simulink library "powerlib_extras"  (Simulink 6.0)
settings: Solver=ode45  SolverMode=SingleTasking  StartTime=0.0  StopTime=10.0  RelTol=1e-3
values from neighbouring files (symbols this model uses):
  Ts = get(handles.edit1,'string')    [powergui.m]
undefined symbols (not defined in the file or in its folder): Ac, Bc, Cc, Dc, Delay_discrete, dend, DiscIntNeverNeededParam, extra_sc, j, numd, test_alpha
libraries: powerlib2 x112, powerlib_extras x70, simulink_extras x25, simulink x12, powerlib_models x8
(part 5 of 9)

== system powerlib_extras/Discrete  Control Blocks/Discrete Monostable ==
  note: Discrete Monostable
  note: Silvano Casoria
      | Power System Simulation Laboratory
      | IREQ, Hydro-Quebc
  In : Inport  Port=1  LatchInput=off
  Constant2 : Constant  Value=-Ts
  Constant3 : Constant  Value=Ts
  Edge_Detector : Subsystem  mask(Discrete Edge Detector){model=EdgeDetect, ic=ic, Ts=Ts}
      mask prompts: model "Edge:"; ic "Input at t = -Ts:"; Ts "Sample time Ts:"
      mask help:
      | This block compares its present input to its previous input.
      |
      | If the input  is a logic signal (TRUE (1) or FALSE (0), the output is a one-step boolean signal TRUE  when  the specified edge (Rising, Falling or Either)  is detected.
      |
      | This block can also be used to detect the slope polarity of a continuous signal. For example, if the specified edge is  "Rising", the output is TRUE as long as the slope of the input signal is positive.
      |
      | The input value at time step preceeding t=0 is specified by the parameter "Input at t=-Ts"
      mask init: same as powerlib_extras/Control  Blocks/Edge Detector
      mask Display: plot(0,0,100,100, X1,Y1,X2,Y2,X3,Y3,X4,Y4);
  Logical Operator1 : Logic
  Logical Operator2 : Logic  Orientation=left  Operator=NOT  Inputs=1
  Relational Operator : RelationalOperator  Operator=>  InputSameDT=on
  Sum1 : Sum  Inputs=+-  SaturateOnIntegerOverflow=on  InputSameDT=on
  Switch : Switch  Threshold=0.5  SaturateOnIntegerOverflow=on  InputSameDT=on
  T_monostable : Constant  Value=t_mono
  Unit Delay : UnitDelay  Orientation=left  SampleTime=Ts
  delay : UnitDelay  Orientation=left  SampleTime=Ts
  Out : Outport
  wires:
  Sum1/1 -> Unit Delay/1, Relational Operator/1
  Unit Delay/1 -> Switch/3
  Constant3/1 -> Sum1/2
  Switch/1 -> Sum1/1
  T_monostable/1 -> Switch/1
  In/1 -> Edge_Detector/1(In)
  Relational Operator/1 -> delay/1, Out/1
  Logical Operator1/1 -> Switch/2
  delay/1 -> Logical Operator2/1
  Logical Operator2/1 -> Logical Operator1/1
  Edge_Detector/1(Out) -> Logical Operator1/2
  Constant2/1 -> Relational Operator/2

== system powerlib_extras/Discrete  Control Blocks/Discrete On/Off Delay ==
  note: Silvano Casoria
      | Power System Simulation Laboratory
      | IREQ, Hydro-Quebc
  note: Discrete On/Off Delay
  IN : Inport  Port=1  LatchInput=off
  Constant : Constant
  Constant1 : Constant  Value=delay
  Constant2 : Constant  Value=type_delay
  Data Type Conversion1 : DataTypeConversion  OutDataTypeMode=boolean  SaturateOnIntegerOverflow=on  RndMeth=Zero
  Logical Operator1 : Logic  Operator=OR
  Logical Operator2 : Logic  Operator=NOT  Inputs=1
  OFF Delay : Subsystem  TreatAsAtomicUnit=on
  ON Delay : Subsystem  TreatAsAtomicUnit=on
  Relational Operator1 : RelationalOperator  Operator===  InputSameDT=on
  OUT : Outport
  wires:
  Data Type Conversion1/1 -> ON Delay/1(IN), OFF Delay/1(IN)
  Constant/1 -> Relational Operator1/2
  Relational Operator1/1 -> ON Delay/Enable, Logical Operator2/1
  Constant2/1 -> Relational Operator1/1
  Logical Operator2/1 -> OFF Delay/Enable
  OFF Delay/1(OUT) -> Logical Operator1/2
  ON Delay/1(OUT) -> Logical Operator1/1
  Logical Operator1/1 -> OUT/1
  Constant1/1 -> ON Delay/2(DELAY), OFF Delay/2(DELAY)
  IN/1 -> Data Type Conversion1/1

== system powerlib_extras/Discrete  Control Blocks/Discrete PI Controller ==
  note: Pierre Giroux, Gilbert Sybille
      | Power System Simulation Laboratory
      | IREQ, Hydro-Quebc
  note: Discrete PID Controller
  Error : Inport  Port=1  LatchInput=off
  Discrete-Time Integrator : DiscreteIntegrator  InitialCondition=Init  SampleTime=Ts  LimitOutput=on  UpperSaturationLimit=UpperLimit  LowerSaturationLimit=LowerLimit  ICPrevOutput=DiscIntNeverNeededParam  ICPrevScaledInput=DiscIntNeverNeededParam
  Kp4 : Gain  Gain=Kp  SaturateOnIntegerOverflow=on
  Kp5 : Gain  Gain=Ki  SaturateOnIntegerOverflow=on
  Saturation2 : Saturate  UpperLimit=UpperLimit  LowerLimit=LowerLimit
  Sum6 : Sum  SaturateOnIntegerOverflow=on  InputSameDT=on
  Out : Outport  InitialOutput=0
  wires:
  Error/1 -> Kp4/1, Kp5/1
  Sum6/1 -> Saturation2/1
  Kp5/1 -> Discrete-Time Integrator/1
  Kp4/1 -> Sum6/1
  Discrete-Time Integrator/1 -> Sum6/2
  Saturation2/1 -> Out/1

== system powerlib_extras/Discrete  Control Blocks/Discrete PID Controller ==
  note: Discrete PID Controller
  note: Pierre Giroux, Gilbert Sybille
      | Power System Simulation Laboratory
      | IREQ, Hydro-Quebc
  Error : Inport  Port=1  LatchInput=off
  "Derivative " : DiscreteTransferFcn  Numerator=[2 -2]  Denominator=[Ts+2*TcD Ts-2*TcD]  SampleTime=Ts
  Discrete-Time Integrator : DiscreteIntegrator  InitialCondition=Init  SampleTime=Ts  LimitOutput=on  UpperSaturationLimit=UpperLimit  LowerSaturationLimit=LowerLimit  ICPrevOutput=DiscIntNeverNeededParam  ICPrevScaledInput=DiscIntNeverNeededParam
  Kp4 : Gain  Gain=Kp  SaturateOnIntegerOverflow=on
  Kp5 : Gain  Gain=Ki  SaturateOnIntegerOverflow=on
  Kp6 : Gain  Gain=Kd  SaturateOnIntegerOverflow=on
  Saturation2 : Saturate  UpperLimit=UpperLimit  LowerLimit=LowerLimit
  Sum6 : Sum  Inputs=+++  SaturateOnIntegerOverflow=on  InputSameDT=on
  Out : Outport  InitialOutput=0
  wires:
  Saturation2/1 -> Out/1
  "Derivative "/1 -> Sum6/3
  Discrete-Time Integrator/1 -> Sum6/2
  Kp4/1 -> Sum6/1
  Kp6/1 -> "Derivative "/1
  Kp5/1 -> Discrete-Time Integrator/1
  Sum6/1 -> Saturation2/1
  Error/1 -> Kp6/1, Kp5/1, Kp4/1

== system powerlib_extras/Discrete  Control Blocks/Discrete PWM Generator ==
  note: PWM Generator
  note: Pierre Giroux, Gilbert Sybille
      | Power System Laboratory, IREQ
      | Hydro-Quebec
  Signal(s) : Inport  Port=1  LatchInput=off
  BL4 : Logic  Operator=NOT  Inputs=1
  BL5 : Logic  Operator=NOT  Inputs=1
  Constant : Constant  Value=Internal_Phase
  Constant1 : Constant  Value=Internal
  Data Type  Conversion : DataTypeConversion  Orientation=down  OutDataTypeMode=double  SaturateOnIntegerOverflow=on  RndMeth=Zero
  Data Type  Conversion1 : DataTypeConversion  OutDataTypeMode=boolean  SaturateOnIntegerOverflow=on  RndMeth=Zero
  Data Type  Conversion2 : DataTypeConversion  OutDataTypeMode=boolean  SaturateOnIntegerOverflow=on  RndMeth=Zero
  Gain : Gain  Gain=2*pi*Freq  SaturateOnIntegerOverflow=on
  Gain2 : Gain  Gain=pi/180  SaturateOnIntegerOverflow=on
  Gain3 : Gain  Gain=-1  SaturateOnIntegerOverflow=on
  Mux : Mux  Inputs=2
  Mux1 : Mux  Inputs=2
  Mux2 : Mux  Inputs=2
  Product : Product  SaturateOnIntegerOverflow=on  InputSameDT=on
  Relational Operator : RelationalOperator  InputSameDT=on
  Relational Operator1 : RelationalOperator  InputSameDT=on
  Select1A : Selector  Elements=Select1_Elements  InputPortWidth=Select1_PortWidth
  Select1B : Selector  Elements=Select1_Elements  InputPortWidth=Select1_PortWidth
  Select3 : Selector  Elements=Select3_Elements  InputPortWidth=Select3_PortWidth
  Sum : Sum  Inputs=+++  SaturateOnIntegerOverflow=on  InputSameDT=on
  Switch : Switch  Threshold=0.5  SaturateOnIntegerOverflow=on  InputSameDT=on
  Triangle : simulink/Sources/Repeating Sequence  rep_seq_t=[0 1/Fc/4 3/Fc/4 1/Fc]  rep_seq_y=[0 -1 1 0]
  Trigonometric Function : Trigonometry
  m3 : Constant  Value=Phase
  m4 : Constant  Value=mIndex
  t : DigitalClock  SampleTime=Ts
  Pulses : Outport
  wires:
  Data Type  Conversion2/1 -> Mux1/1, BL5/1
  Relational Operator1/1 -> Data Type  Conversion2/1
  Data Type  Conversion1/1 -> Mux/1, BL4/1
  Relational Operator/1 -> Data Type  Conversion1/1
  Data Type  Conversion/1 -> Pulses/1
  Select3/1 -> Data Type  Conversion/1
  t/1 -> Gain/1
  Gain/1 -> Sum/1
  Gain2/1 -> Sum/2
  m3/1 -> Gain2/1
  Constant/1 -> Sum/3
  m4/1 -> Product/1
  Sum/1 -> Trigonometric Function/1
  Trigonometric Function/1 -> Product/2
  Signal(s)/1 -> Switch/3
  Constant1/1 -> Switch/2
  Product/1 -> Switch/1
  Triangle/1 -> Relational Operator/2, Relational Operator1/2
  Gain3/1 -> Relational Operator1/1
  BL4/1 -> Mux/2
  BL5/1 -> Mux1/2
  Mux/1 -> Select1A/1
  Mux1/1 -> Select1B/1
  Select1A/1 -> Mux2/1
  Select1B/1 -> Mux2/2
  Mux2/1 -> Select3/1
  Switch/1 -> Gain3/1, Relational Operator/1

== system powerlib_extras/Discrete  Control Blocks/Discrete Rate Limiter ==
  note: Delta(u)
  note: Beat Ronner
      | ABB Industrie AG
      | Turgi, Switzerland
  In : Inport  Port=1  LatchInput=off
  Saturation : Saturate  UpperLimit=UpperLimit  LowerLimit=LowerLimit
  Sum : Sum  Inputs=|++  SaturateOnIntegerOverflow=on  InputSameDT=on
  Sum1 : Sum  Inputs=|+-  SaturateOnIntegerOverflow=on  InputSameDT=on
  Unit  Delay : UnitDelay  Orientation=left  X0=Vinit  SampleTime=Ts
  Out : Outport
  wires:
  In/1 -> Sum1/1  "u"
  Sum1/1 -> Saturation/1
  Saturation/1 -> Sum/1  "Delta(u)_limit"
  Sum/1 -> Out/1, Unit  Delay/1  "y"
  Unit  Delay/1 -> Sum1/2, Sum/2  "y-1"

== system powerlib_extras/Discrete  Control Blocks/Discrete Sample & Hold ==
  note: Sample and Hold
  note: Silvano Casoria
      | Power System Simulation Laboratory
      | IREQ, Hydro-Quebc
  In : Inport  Port=1  LatchInput=off
  S : Inport  Port=2  LatchInput=off
  Switch : Switch  Threshold=0.5  SaturateOnIntegerOverflow=on  InputSameDT=on
  Unit Delay : UnitDelay  Orientation=left  X0=ic  SampleTime=Ts
  "   " : Outport  InitialOutput=0
  wires:
  Switch/1 -> Unit Delay/1, "   "/1
  Unit Delay/1 -> Switch/3
  In/1 -> Switch/1
  S/1 -> Switch/2

== system powerlib_extras/Discrete  Control Blocks/Discrete Shift Register ==
  u(k) : Inport  Port=1  LatchInput=off
  "S-Function " : S-Function  FunctionName=discreteNLastSamples  Parameters=NSamples,Ts,InitialValue
  Out : Outport
  wires:
  "S-Function "/1 -> Out/1
  u(k)/1 -> "S-Function "/1

== system powerlib_extras/Discrete  Control Blocks/Discrete Virtual PLL ==
  note: Discrete Virtual PLL
  note: Pierre Giroux, Gilbert Sybille
      | Power System Simulation Laboratory
      | IREQ, Hydro-Quebc
  Constant4 : Constant  Value=2*pi
  Deg->Rad : Gain  Gain=pi/180  SaturateOnIntegerOverflow=on
  Freq1 : Constant  Value=Freq
  Freq2 : Constant  Value=2*pi
  Initial Vd_Vq1 : Constant  Value=Phase
  Math Function : Math  Operator=mod  SaturateOnIntegerOverflow=on
  Mux : Mux  Inputs=2
  Product : Product  Inputs=***  SaturateOnIntegerOverflow=on  InputSameDT=on
  Sum : Sum  SaturateOnIntegerOverflow=on  InputSameDT=on
  Trigonometric Function : Trigonometry
  Trigonometric Function1 : Trigonometry  Operator=cos
  t : DigitalClock  SampleTime=Ts
  Freq : Outport
  Sin_Cos : Outport  Port=2
  wt : Outport  Port=3
  wires:
  Mux/1 -> Sin_Cos/1
  Trigonometric Function1/1 -> Mux/2
  Trigonometric Function/1 -> Mux/1
  Math Function/1 -> Trigonometric Function/1, Trigonometric Function1/1, wt/1
  Constant4/1 -> Math Function/2
  Product/1 -> Sum/1
  Initial Vd_Vq1/1 -> Deg->Rad/1
  Deg->Rad/1 -> Sum/2
  Freq1/1 -> Freq/1, Product/1
  Freq2/1 -> Product/3
  t/1 -> Product/2
  Sum/1 -> Math Function/1

== system powerlib_extras/Discrete  Control Blocks/Discrete  2nd-Order Filter ==
  In : Inport  Port=1  LatchInput=off
  Discrete State-Space : DiscreteStateSpace  A=Ad  B=Bd  C=Cd  D=Dd  X0=x0d  SampleTime=Ts
  Out : Outport  InitialOutput=0
  wires:
  In/1 -> Discrete State-Space/1
  Discrete State-Space/1 -> Out/1

== system powerlib_extras/Discrete  Control Blocks/Discrete  Butterworth Filter  ==
  In : Inport  Port=1  LatchInput=off
  Discrete State-Space : DiscreteStateSpace  A=Ad  B=Bd  C=Cd  D=Dd  X0=x0d  SampleTime=Ts
  Out : Outport  InitialOutput=0
  wires:
  In/1 -> Discrete State-Space/1
  Discrete State-Space/1 -> Out/1

== system powerlib_extras/Discrete  Control Blocks/Discrete 12-Pulse HVDC Control  ==
  note: Silvano Casoria
      | (Rev. 2001)
      | Power System Laboratory, IREQ
      | Hydro-Quebec
  note: Note 2 : gamma control is not implemented
  note: Note 1 : PLL is not simulated ; a fixed frequency is assumed
  note: Rect = 0
      | Inverter = 1
  note: 12-PULSE HVDC CONTROL
  Vabc (pu) : Inport  Port=1  LatchInput=off
  VdL (pu) : Inport  Port=2  LatchInput=off
  Id (pu) : Inport  Port=3  LatchInput=off
  Id_ref (pu) : Inport  Port=4  LatchInput=off
  Vd_ref (pu) : Inport  Port=5  LatchInput=off
  Block : Inport  Port=6  LatchInput=off
  ForcedAlpha : Inport  Port=7  LatchInput=off
  2nd order BP filters : Subsystem
  Alpha Control : Subsystem  mask{test_alpha=test_alpha, alpha_fix=alpha_fix}
      mask prompts: test_alpha "alpha control (0=normal; 1=constant alpha)"; alpha_fix "Constant alpha value (degrees) :"
  Demux : Demux  Outputs=3
  Discrete Synchronized 12-Pulse Generator : powerlib_extras/Discrete  Control Blocks/Discrete Synchronized 12-Pulse Generator  pwidth=Pw  Double_Pulse=off  Ts=pas
  Freq : Constant  Value=f0
  Functions (Discrete) : Subsystem
  "Parameter  Selection " : Subsystem
  alpha_min_inv (deg) : Constant  Value=Mode - 1
  PulsesY : Outport
  PulsesD : Outport  Port=2
  alpha (deg) : Outport  Port=3
  Id_ref_lim (pu) : Outport  Port=4
  Mode : Outport  Port=5
  wires:
  ForcedAlpha/1 -> Alpha Control/3(forced delay)
  Functions (Discrete)/3(mode) -> Mode/1
  Freq/1 -> Discrete Synchronized 12-Pulse Generator/5
  Discrete Synchronized 12-Pulse Generator/1 -> PulsesY/1
  Discrete Synchronized 12-Pulse Generator/2 -> PulsesD/1
  Block/1 -> Functions (Discrete)/12(Block), Discrete Synchronized 12-Pulse Generator/6
  Demux/2 -> 2nd order BP filters/2(B)
  Alpha Control/2(min_i) -> Functions (Discrete)/8(Min_i)
  Alpha Control/1(max_i) -> Functions (Discrete)/7(Max_i)
  Functions (Discrete)/2(Id_ref_lim) -> Id_ref_lim (pu)/1
  Demux/3 -> 2nd order BP filters/3(C)
  Demux/1 -> 2nd order BP filters/1(A)
  "Parameter  Selection "/6(min_lin) -> Functions (Discrete)/10(min_lin)
  "Parameter  Selection "/5(max_lin) -> Functions (Discrete)/9(max_lin)
  "Parameter  Selection "/2(Vd_marg) -> Functions (Discrete)/6(Vd_marg)
  "Parameter  Selection "/1(Id_marg) -> Functions (Discrete)/5(Id_marg)
  Id (pu)/1 -> Functions (Discrete)/3(Id (pu))
  VdL (pu)/1 -> Functions (Discrete)/1(VdL (pu))
  Id_ref (pu)/1 -> Functions (Discrete)/4(Id_ref (pu))
  Vd_ref (pu)/1 -> Functions (Discrete)/2(Vd_ref (pu))
  2nd order BP filters/1("A ") -> Discrete Synchronized 12-Pulse Generator/2
  2nd order BP filters/2("B ") -> Discrete Synchronized 12-Pulse Generator/3
  2nd order BP filters/3("C ") -> Discrete Synchronized 12-Pulse Generator/4
  Functions (Discrete)/1(Alpha_ord) -> alpha (deg)/1, Discrete Synchronized 12-Pulse Generator/1
  "Parameter  Selection "/4(alpha_min) -> Alpha Control/2(alpha_min)
  "Parameter  Selection "/3(alpha_max) -> Alpha Control/1(alpha_max)
  alpha_min_inv (deg)/1 -> Functions (Discrete)/11(Inverter), "Parameter  Selection "/1(Inverter)
  Vabc (pu)/1 -> Demux/1

== system powerlib_extras/Discrete  Control Blocks/Discrete 3-phase PWM Generator ==
  note: P.Dahler
      | ABB Industrie AG
  note: (Bridge 1)
  note: (Bridge 2)
  note: 2- or 3-level, 3-phase
      | (single and twin configuration)
      | PWM Modulator
  note: Pierre Giroux, Gilbert Sybille
      | Power System Laboratory, IREQ
      | Hydro-Quebec
  Ust : Inport  Port=1  LatchInput=off
  wt : Inport  Port=2  LatchInput=off
  2-level Type : Subsystem  TreatAsAtomicUnit=on
  3-level Type : Subsystem  TreatAsAtomicUnit=on
  Constant : Constant  Value=2*pi
  Constant2 : Constant  Value=ModulatorType
  Constant3 : Constant  Value=Fc
  Constant4 : Constant  Value=ModulatorMode
  Constant5 : Constant  Value=CmdModulatingSignals
  Constant6 : Constant
  Gain4 : Gain  Gain=nF  SaturateOnIntegerOverflow=on
  Internal : Subsystem  mask(3-ph signal generator){m=m, Freq=Freq, Phase=Phase, Ts=Ts}
      mask prompts: m "Modulation Index:"; Freq "Output signal frequency (Hz):"; Phase "Output signal phase (degrees):"; Ts "Sample time:"
  Logical Operator : Logic  Operator=NOT
  Multiport Switch : MultiPortSwitch  Inputs=2  InputSameDT=on
  Multiport Switch1 : MultiPortSwitch  Inputs=2  InputSameDT=on
  Product : Product  Inputs=3  SaturateOnIntegerOverflow=on  InputSameDT=on
  Relational Operator : RelationalOperator  Operator===  InputSameDT=on
  Select 2- or 3-level : Subsystem
  SubSystem : Subsystem
      mask Display: disp('Pulse pattern\ndescription')
  t : DigitalClock  SampleTime=Ts
  P1 : Outport
  P2 : Outport  Port=2
  wires:
  2-level Type/2(P2) -> Select 2- or 3-level/3(P2 (2-L))
  2-level Type/1(P1) -> Select 2- or 3-level/2(P1 (2-L))
  Select 2- or 3-level/1(P1) -> P1/1
  Select 2- or 3-level/2(P2) -> P2/1
  3-level Type/2(P2) -> Select 2- or 3-level/5(P2 (3-L))
  3-level Type/1(P1) -> Select 2- or 3-level/4(P1 (3-L))
  Logical Operator/1 -> Select 2- or 3-level/1(Select), 3-level Type/Enable
  Constant2/1 -> Relational Operator/1
  Relational Operator/1 -> Logical Operator/1, 2-level Type/Enable
  Constant6/1 -> Relational Operator/2
  Multiport Switch1/1 -> 3-level Type/1(Ust), 2-level Type/1(Ust)  "Ust (3 ph)"
  Multiport Switch/1 -> 3-level Type/2(wt), 2-level Type/2(wt)
  Constant/1 -> Product/1
  Constant3/1 -> Product/2
  t/1 -> Product/3
  wt/1 -> Gain4/1
  Constant4/1 -> Multiport Switch/1
  Gain4/1 -> Multiport Switch/2
  Product/1 -> Multiport Switch/3
  Internal/1("Ust ") -> Multiport Switch1/3
  Constant5/1 -> Multiport Switch1/1
  Ust/1 -> Multiport Switch1/2

== system powerlib_extras/Discrete  Control Blocks/Discrete Gamma Measurement ==
  note: Silvano Casoria
      | Power System Simulation Laboratory
      |  IREQ, Hydro-Quebec
  note: Gamma measurement of a six-pulse thyristor bridge
  note: Outgoing  Conducting      Commutation Voltage (Uak)
      | Valve         Valves                Y          D1(lag)     D11(lead)
      | ---------      ----------------     --------   ------------    -------------
      |     1                 2-3                Uab         Ua              -Ub
      |     2                 3-4                Uac        -Uc                Ua
      |     3                 4-5                Ubc         Ub              -Uc
      |     4                 5-6                Uba       -Ua                Ub
      |     5                 6-1                Uca         Uc              -Ua
      |     6                 1-2                Ucb        -Ub               Uc
  I_th(1-6) : Inport  Port=1  LatchInput=off
  Uabc : Inport  Port=2  LatchInput=off
  Freq : Inport  Port=3  LatchInput=off
  Clock : Clock
      settings: Decimation=10
  Commutation Voltages : Subsystem
  Discrete Bistable : powerlib_extras/Discrete  Control Blocks/Discrete Bistable  Priority=667390432  ic=0  Ts=Ts
  Discrete Edge Detector : powerlib_extras/Discrete  Control Blocks/Discrete Edge Detector  model=Rising  ic=0  Ts=Ts
  Discrete Edge Detector1 : powerlib_extras/Discrete  Control Blocks/Discrete Edge Detector  model=Rising  ic=0  Ts=Ts
  Discrete Monostable : powerlib_extras/Discrete  Control Blocks/Discrete Monostable  EdgeDetect=Rising  t_mono=4/(360*f0)  ic=0  Ts=Ts
  Discrete Monostable1 : powerlib_extras/Discrete  Control Blocks/Discrete Monostable  EdgeDetect=Rising  t_mono=86/(360*f0)  ic=0  Ts=Ts
  Discrete Sample & Hold : powerlib_extras/Discrete  Control Blocks/Discrete Sample & Hold  ic=0  Ts=Ts
  Discrete Sample & Hold1 : powerlib_extras/Discrete  Control Blocks/Discrete Sample & Hold  ic=0  Ts=Ts
  Discrete Sample & Hold2 : powerlib_extras/Discrete  Control Blocks/Discrete Sample & Hold  ic=0  Ts=Ts
  Gain1 : Gain  Gain=60  SaturateOnIntegerOverflow=on
  Gain2 : Gain  Gain=360  SaturateOnIntegerOverflow=on
  Gain7 : Gain  Gain=-1  SaturateOnIntegerOverflow=on
  Hit  (Falling) : HitCross  HitCrossingOffset=Ith_min  HitCrossingDirection=falling
  "Hit  (Falling) " : HitCross  HitCrossingDirection=falling
  MinMax1 : MinMax  SaturateOnIntegerOverflow=on  InputSameDT=on
  Product : Product  SaturateOnIntegerOverflow=on
  Product1 : Product  SaturateOnIntegerOverflow=on
  Sum : Sum  Inputs=|-+  SaturateOnIntegerOverflow=on  InputSameDT=on
  Sum1 : Sum  Inputs=+  SaturateOnIntegerOverflow=on  InputSameDT=on
  gamma_min (deg) : Outport
  gamma_mean (deg) : Outport  Port=2
  Ucom(1-6) : Outport  Port=3
  wires:
  Product/1 -> gamma_mean (deg)/1
  Sum1/1 -> Product/1
  Discrete Sample & Hold2/1 -> Sum1/1, MinMax1/1  "t_gamma"
  Discrete Edge Detector1/1 -> Discrete Sample & Hold/2, Discrete Sample & Hold2/2
  Product1/1 -> gamma_min (deg)/1
  MinMax1/1 -> Product1/1
  Discrete Sample & Hold/1 -> Sum/2  "t1"
  Sum/1 -> Discrete Sample & Hold2/1
  Discrete Bistable/1 -> Discrete Edge Detector/1
  Discrete Edge Detector/1 -> Discrete Sample & Hold1/2
  I_th(1-6)/1 -> Hit  (Falling)/1
  Hit  (Falling)/1 -> Discrete Monostable/1
  "Hit  (Falling) "/1 -> Discrete Monostable1/1
  Discrete Monostable/1 -> Discrete Bistable/1
  Discrete Monostable1/1 -> Discrete Bistable/2
  Discrete Bistable/2 -> Discrete Edge Detector1/1
  Clock/1 -> Discrete Sample & Hold/1, Discrete Sample & Hold1/1
  Discrete Sample & Hold1/1 -> Sum/1  "t0"
  Gain7/1 -> "Hit  (Falling) "/1
  Commutation Voltages/1(Ucom (1-6)) -> Gain7/1, Ucom(1-6)/1
  Uabc/1 -> Commutation Voltages/1(Uabc)  "Ua Ub Uc"
  Gain1/1 -> Product/2
  Freq/1 -> Gain1/1, Gain2/1
  Gain2/1 -> Product1/2

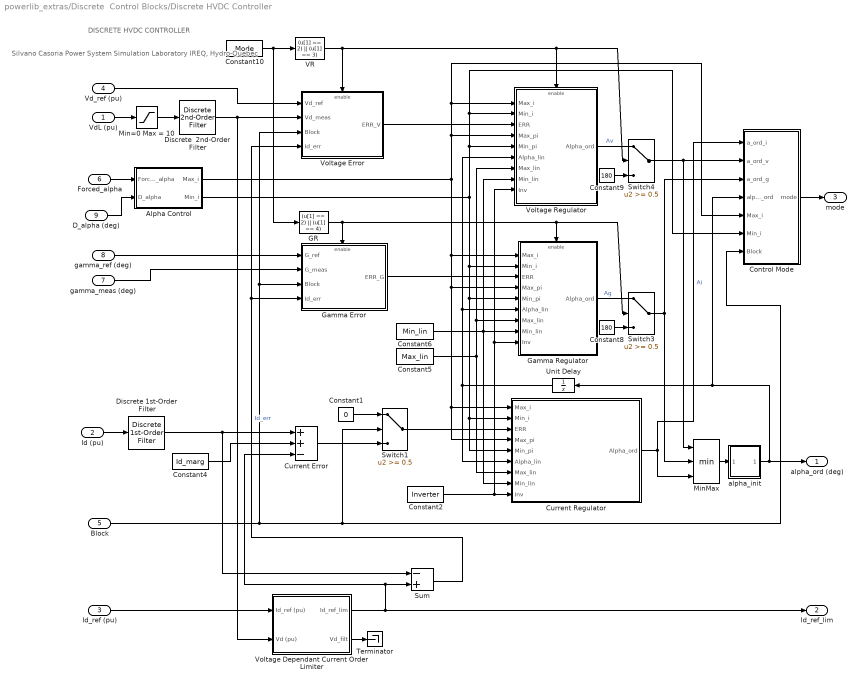
== system powerlib_extras/Discrete  Control Blocks/Discrete HVDC Controller ==
  note: Silvano Casoria
      | Power System Simulation Laboratory
      |  IREQ, Hydro-Quebec
  note: DISCRETE HVDC CONTROLLER
  VdL (pu) : Inport  Port=1  LatchInput=off
  Id (pu) : Inport  Port=2  LatchInput=off
  Id_ref (pu) : Inport  Port=3  LatchInput=off
  Vd_ref (pu) : Inport  Port=4  LatchInput=off
  Block : Inport  Port=5  LatchInput=off
  Forced_alpha : Inport  Port=6  LatchInput=off
  gamma_meas (deg) : Inport  Port=7  LatchInput=off
  gamma_ref (deg) : Inport  Port=8  LatchInput=off
  D_alpha (deg) : Inport  Port=9  LatchInput=off
  Alpha Control : Subsystem
  Constant1 : Constant  Value=0
  Constant10 : Constant  Value=Mode
  Constant2 : Constant  Value=Inverter
  Constant4 : Constant  Value=Id_marg
  Constant5 : Constant  Value=Max_lin
  Constant6 : Constant  Value=Min_lin
  Constant8 : Constant  Value=180
  Constant9 : Constant  Value=180
  "Control Mode " : Subsystem
  Current Error : Sum  Inputs=++-  SaturateOnIntegerOverflow=on  InputSameDT=on
  Current Regulator : Subsystem  mask(PI Regulator  With  External  Limits (Discrete)){Kp=Kp_I, Ki=Ki_I, IC_i=ICi_I, On_lin=on, dt=dt}
      mask prompts: Kp "Kp (deg/pu):"; Ki "Ki (deg/pu/s):"; IC_i "Integrator Initial Condition (deg):"; On_lin "Linearization  (On)"; dt "Sample time (s):"
      mask help: For the linearization it is important to specifie the mode of operation i.e. rectifier or inverter (negation of rectifier).
      mask Display: disp('PI Regulator\nWith external limits\n(Linearized Kp)\n(Discrete)\n\n')
  Discrete 1st-Order Filter : powerlib_extras/Discrete  Control Blocks/Discrete 1st-Order Filter  FilterType=Lowpass  Tc=T_I  Ts=dt  Initialize=off  Vac_Init=[0.8 -25 60]  Vdc_Init=-0.4  PlotResponse=off  param1=[1 500 0.1]
  Discrete  2nd-Order Filter : powerlib_extras/Discrete  Control Blocks/Discrete  2nd-Order Filter  FilterType=Lowpass  Fo=f0_V  Zeta=Z_V  Ts=dt  Initialize=off  Vac_Init=[0.8 -25 60]  Vdc_Init=-0.4  PlotResponse=off  param1=[1 500 1]
  GR : Fcn  Expr=(u[1] == 2) || (u[1] == 4)
  Gamma Error : Subsystem  TreatAsAtomicUnit=on
  Gamma Regulator : Subsystem  TreatAsAtomicUnit=on
  Min=0 Max = 10 : Saturate  UpperLimit=10  LowerLimit=0
  MinMax : MinMax  Inputs=3  SaturateOnIntegerOverflow=on  InputSameDT=on
  Sum : Sum  Inputs=-+  SaturateOnIntegerOverflow=on  InputSameDT=on
  Switch1 : Switch  Threshold=0.5  SaturateOnIntegerOverflow=on  InputSameDT=on
  Switch3 : Switch  Threshold=0.5  SaturateOnIntegerOverflow=on  InputSameDT=on
  Switch4 : Switch  Threshold=0.5  SaturateOnIntegerOverflow=on  InputSameDT=on
  Terminator : Terminator
  Unit Delay : UnitDelay  Orientation=left  SampleTime=dt
  VR : Fcn  Expr=(u[1] == 2) || (u[1] == 3)
  Voltage Dependant Current Order Limiter : Subsystem  mask(Voltage Dependent Current Order Limiter  (Discrete)){Vd_seuil=Vd_seuil, Vd_min=Vd_min, Id_min=Id_min, Id_min_abs=Id_min_abs, Tu=Tup, pas=dt}
      mask prompts: Vd_seuil "Vd seuil (pu):"; Vd_min "Vd min (pu):"; Id_min "Id min (pu):"; Id_min_abs "Id min abs (pu):"; Tu "Up Time constant (s):"; pas "Sample time (s):"
      mask Display: disp('VDCOL\n (Discrete)')
  Voltage Error : Subsystem  TreatAsAtomicUnit=on
  Voltage Regulator : Subsystem  TreatAsAtomicUnit=on
  alpha_init : Subsystem
  alpha_ord (deg) : Outport
  Id_ref_lim : Outport  Port=2
  mode : Outport  Port=3
  wires:
  Forced_alpha/1 -> Alpha Control/1(Forced_alpha)
  "Control Mode "/1(mode) -> mode/1
  Voltage Error/1(ERR_V) -> Voltage Regulator/3(ERR)
  Vd_ref (pu)/1 -> Voltage Error/1(Vd_ref)
  Sum/1 -> Gamma Error/4(Id_err), Voltage Error/4(Id_err)  "Id_err"
  gamma_meas (deg)/1 -> Gamma Error/2(G_meas)
  gamma_ref (deg)/1 -> Gamma Error/1(G_ref)
  Gamma Error/1(ERR_G) -> Gamma Regulator/3(ERR)
  Constant1/1 -> Switch1/1
  Switch4/1 -> "Control Mode "/2(a_ord_v), MinMax/1
  Switch3/1 -> "Control Mode "/3(a_ord_g), MinMax/2
  Current Regulator/1(Alpha_ord) -> "Control Mode "/1("a_ord_i "), MinMax/3  "Ai"
  Constant9/1 -> Switch4/3
  Voltage Regulator/1(Alpha_ord) -> Switch4/1  "Av"
  Constant8/1 -> Switch3/3
  Gamma Regulator/1(Alpha_ord) -> Switch3/1  "Ag"
  Switch1/1 -> Current Regulator/3(ERR)
  Constant2/1 -> Current Regulator/9(Inv), Gamma Regulator/9(Inv), Voltage Regulator/9(Inv)
  Block/1 -> Voltage Error/3(Block), Gamma Error/3(Block), "Control Mode "/7(Block), Switch1/2
  Alpha Control/2(Min_i) -> Voltage Regulator/5(Min_pi), "Control Mode "/6(Min_i), Voltage Regulator/2(Min_i), Gamma Regulator/2(Min_i), Gamma Regulator/5(Min_pi), Current Regulator/2(Min_i), Current Regulator/5(Min_pi)
  Constant5/1 -> Current Regulator/7(Max_lin), Voltage Regulator/7(Max_lin), Gamma Regulator/7(Max_lin)
  alpha_init/1(Out1) -> "Control Mode "/4(alpha_ord), Unit Delay/1, alpha_ord (deg)/1
  Unit Delay/1 -> Current Regulator/6(Alpha_lin), Voltage Regulator/6(Alpha_lin), Gamma Regulator/6(Alpha_lin)
  MinMax/1 -> alpha_init/1(In1)
  Current Error/1 -> Switch1/3
  Discrete 1st-Order Filter/1 -> Current Error/1, Sum/1
  Id (pu)/1 -> Discrete 1st-Order Filter/1
  VdL (pu)/1 -> Min=0 Max = 10/1
  Min=0 Max = 10/1 -> Discrete  2nd-Order Filter/1
  Discrete  2nd-Order Filter/1 -> Voltage Error/2(Vd_meas), Voltage Dependant Current Order Limiter/2(Vd (pu))
  Voltage Dependant Current Order Limiter/1(Id_ref_lim) -> Current Error/3, Sum/2, Id_ref_lim/1
  Voltage Dependant Current Order Limiter/2(Vd_filt) -> Terminator/1
  Id_ref (pu)/1 -> Voltage Dependant Current Order Limiter/1(Id_ref (pu))
  Constant4/1 -> Current Error/2
  Constant6/1 -> Current Regulator/8(Min_lin), Voltage Regulator/8(Min_lin), Gamma Regulator/8(Min_lin)
  Alpha Control/1(Max_i) -> Voltage Regulator/4(Max_pi), "Control Mode "/5(Max_i), Voltage Regulator/1(Max_i), Gamma Regulator/1(Max_i), Gamma Regulator/4(Max_pi), Current Regulator/1(Max_i), Current Regulator/4(Max_pi)
  D_alpha (deg)/1 -> Alpha Control/2(D_alpha)
  VR/1 -> Voltage Regulator/Enable, Switch4/2, Voltage Error/Enable
  Constant10/1 -> GR/1, VR/1
  GR/1 -> Gamma Regulator/Enable, Switch3/2, Gamma Error/Enable

== system powerlib_extras/Discrete  Control Blocks/Discrete SV PWM Generator ==
  note: Hoang Le-Huy
      | Universite Laval
      | Quebec
  note: Pierre Giroux, Gilbert Sybille
      | Power System Laboratory, IREQ
      | Hydro-Quebec
  note: Space Vector Pulse Width Modulation (SV PWM)
  Umag : Inport  Port=1  LatchInput=off
  Uangle : Inport  Port=2  LatchInput=off
  Constant : Constant
  Constant1 : Constant  Value=Freq
  Constant2 : Constant  Value=m
  Constant3 : Constant  Value=Pha
  Constant4 : Constant  Value=SwitchingPattern
  Determine reference vector (U*) : Subsystem
  INFO : Subsystem
      mask Display: disp('?')
  Logical Operator : Logic  Orientation=down  Operator=NOT  AllPortsSameDT=off
  Multiport Switch : MultiPortSwitch  Inputs=2  SaturateOnIntegerOverflow=on
  Relational Operator : RelationalOperator  Operator===
  SV Modulator Pattern #1 : Subsystem
  SV Modulator Pattern #2 : Subsystem
  Pulses : Outport
  wires:
  Logical Operator/1 -> SV Modulator Pattern #2/Enable
  Relational Operator/1 -> Logical Operator/1, SV Modulator Pattern #1/Enable
  Constant/1 -> Relational Operator/2
  Constant4/1 -> Relational Operator/1, Multiport Switch/1
  Constant3/1 -> Determine reference vector (U*)/5(Pha_Init)
  Constant1/1 -> Determine reference vector (U*)/4(Freq_Int)
  Constant2/1 -> Determine reference vector (U*)/3(m_Int)
  Determine reference vector (U*)/2(alpha) -> SV Modulator Pattern #1/2(alpha), SV Modulator Pattern #2/2(alpha)
  Determine reference vector (U*)/1(m) -> SV Modulator Pattern #1/1(m), SV Modulator Pattern #2/1(m)
  Multiport Switch/1 -> Pulses/1
  SV Modulator Pattern #2/1(Pulses) -> Multiport Switch/3
  SV Modulator Pattern #1/1(Pulses) -> Multiport Switch/2
  Uangle/1 -> Determine reference vector (U*)/2(In2)
  Umag/1 -> Determine reference vector (U*)/1(In1)

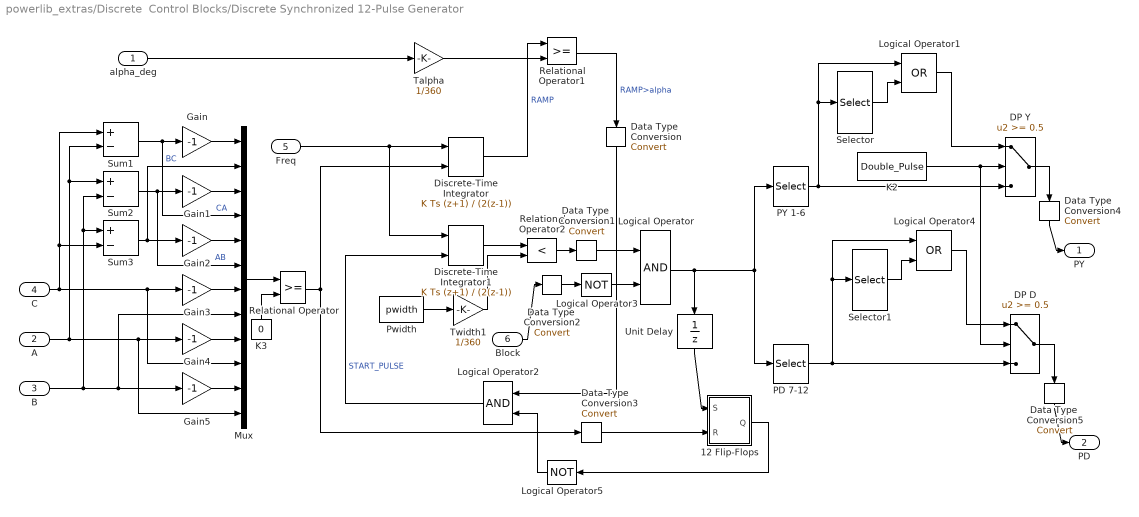
== system powerlib_extras/Discrete  Control Blocks/Discrete Synchronized 12-Pulse Generator ==
  alpha_deg : Inport  Port=1  LatchInput=off
  A : Inport  Port=2  LatchInput=off
  B : Inport  Port=3  LatchInput=off
  C : Inport  Port=4  LatchInput=off
  Freq : Inport  Port=5  LatchInput=off
  Block : Inport  Port=6  LatchInput=off
  12 Flip-Flops : Subsystem
  DP D : Switch  Threshold=0.5  InputSameDT=on
  DP Y : Switch  Threshold=0.5  InputSameDT=on
  Data Type  Conversion : DataTypeConversion  Orientation=down  OutDataTypeMode=boolean  SaturateOnIntegerOverflow=on  RndMeth=Zero
  Data Type  Conversion1 : DataTypeConversion  OutDataTypeMode=boolean  SaturateOnIntegerOverflow=on  RndMeth=Zero
  Data Type  Conversion2 : DataTypeConversion  OutDataTypeMode=boolean  SaturateOnIntegerOverflow=on  RndMeth=Zero
  Data Type  Conversion3 : DataTypeConversion  OutDataTypeMode=boolean  SaturateOnIntegerOverflow=on  RndMeth=Zero
  Data Type  Conversion4 : DataTypeConversion  Orientation=down  OutDataTypeMode=double  SaturateOnIntegerOverflow=on  RndMeth=Zero
  Data Type  Conversion5 : DataTypeConversion  Orientation=down  OutDataTypeMode=double  SaturateOnIntegerOverflow=on  RndMeth=Zero
  Discrete-Time Integrator : DiscreteIntegrator  IntegratorMethod=Integration: Trapezoidal  ExternalReset=rising  SampleTime=Ts  ICPrevOutput=DiscIntNeverNeededParam  ICPrevScaledInput=DiscIntNeverNeededParam
  Discrete-Time Integrator1 : DiscreteIntegrator  IntegratorMethod=Integration: Trapezoidal  ExternalReset=rising  SampleTime=Ts  ICPrevOutput=DiscIntNeverNeededParam  ICPrevScaledInput=DiscIntNeverNeededParam
  Gain{,1..5} (6 alike) : Gain  Gain=-1  SaturateOnIntegerOverflow=on
  K2 : Constant  Value=Double_Pulse
  K3 : Constant  Orientation=up  Value=0
  Logical Operator : Logic
  Logical Operator1 : Logic  Operator=OR
  Logical Operator2 : Logic  Orientation=left
  Logical Operator3 : Logic  Operator=NOT  Inputs=1
  Logical Operator4 : Logic  Operator=OR
  Logical Operator5 : Logic  Orientation=left  Operator=NOT  Inputs=1
  Mux : Mux  Inputs=12
  PD 7-12 : Selector  Elements=7:12  InputPortWidth=12
  PY 1-6 : Selector  Elements=1:6  InputPortWidth=12
  Pwidth : Constant  Value=pwidth
  Relational Operator : RelationalOperator  InputSameDT=on
  Relational Operator1 : RelationalOperator  InputSameDT=on
  Relational Operator2 : RelationalOperator  Operator=<  InputSameDT=on
  Selector : Selector  Elements=[2 3 4 5 6 1 ]  InputPortWidth=6
  Selector1 : Selector  Elements=[2 3 4 5 6 1 ]  InputPortWidth=6
  Sum1 : Sum  Inputs=+-  SaturateOnIntegerOverflow=on  InputSameDT=on
  Sum2 : Sum  Inputs=+-  SaturateOnIntegerOverflow=on  InputSameDT=on
  Sum3 : Sum  Inputs=+-  SaturateOnIntegerOverflow=on  InputSameDT=on
  Talpha : Gain  Gain=1/360  SaturateOnIntegerOverflow=on
  Twidth1 : Gain  Gain=1/360  SaturateOnIntegerOverflow=on
  Unit Delay : UnitDelay  Orientation=down  SampleTime=Ts
  PY : Outport  InitialOutput=0
  PD : Outport  Port=2  InitialOutput=0
  wires:
  Freq/1 -> Discrete-Time Integrator1/1, Discrete-Time Integrator/1
  K3/1 -> Relational Operator/2
  Mux/1 -> Relational Operator/1
  Gain2/1 -> Mux/5
  Gain1/1 -> Mux/3
  Gain/1 -> Mux/1
  alpha_deg/1 -> Talpha/1
  Sum1/1 -> Gain/1, Mux/4  "CA"
  Sum2/1 -> Gain1/1, Mux/6  "AB"
  Sum3/1 -> Gain2/1, Mux/2  "BC"
  Gain3/1 -> Mux/7
  Gain4/1 -> Mux/9
  Gain5/1 -> Mux/11
  C/1 -> Gain3/1, Mux/10, Sum1/1, Sum3/2
  A/1 -> Gain4/1, Mux/12, Sum2/1, Sum1/2
  B/1 -> Gain5/1, Mux/8, Sum3/1, Sum2/2
  Discrete-Time Integrator/1 -> Relational Operator1/1  "RAMP"
  Talpha/1 -> Relational Operator1/2
  Discrete-Time Integrator1/1 -> Relational Operator2/1
  Twidth1/1 -> Relational Operator2/2
  Logical Operator2/1 -> Discrete-Time Integrator1/2  "START_PULSE"
  Logical Operator5/1 -> Logical Operator2/2
  Relational Operator/1 -> Discrete-Time Integrator/2, Data Type  Conversion3/1
  Pwidth/1 -> Twidth1/1
  Logical Operator3/1 -> Logical Operator/2
  12 Flip-Flops/1(Q) -> Logical Operator5/1
  Logical Operator/1 -> Unit Delay/1, PY 1-6/1, PD 7-12/1
  Logical Operator1/1 -> DP Y/1
  Selector/1 -> Logical Operator1/2
  PY 1-6/1 -> DP Y/3, Selector/1, Logical Operator1/1
  Logical Operator4/1 -> DP D/1
  Selector1/1 -> Logical Operator4/2
  PD 7-12/1 -> Logical Operator4/1, Selector1/1, DP D/3
  K2/1 -> DP Y/2, DP D/2
  Unit Delay/1 -> 12 Flip-Flops/1(S)
  Relational Operator1/1 -> Data Type  Conversion/1  "RAMP>alpha"
  Data Type  Conversion/1 -> Logical Operator2/1
  Relational Operator2/1 -> Data Type  Conversion1/1
  Data Type  Conversion1/1 -> Logical Operator/1
  Block/1 -> Data Type  Conversion2/1
  Data Type  Conversion2/1 -> Logical Operator3/1
  Data Type  Conversion3/1 -> 12 Flip-Flops/2(R)
  DP Y/1 -> Data Type  Conversion4/1
  Data Type  Conversion4/1 -> PY/1
  DP D/1 -> Data Type  Conversion5/1
  Data Type  Conversion5/1 -> PD/1

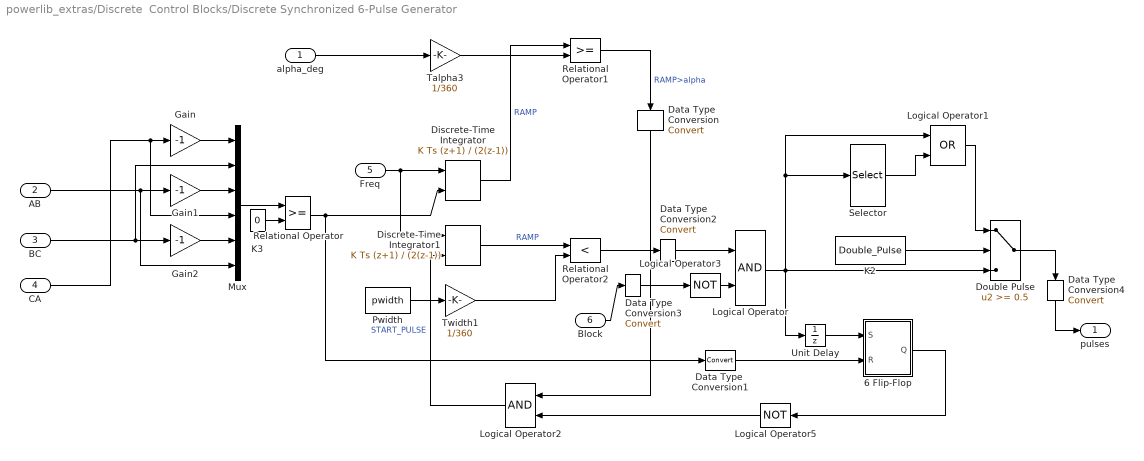
== system powerlib_extras/Discrete  Control Blocks/Discrete Synchronized 6-Pulse Generator ==
  alpha_deg : Inport  Port=1  LatchInput=off
  AB : Inport  Port=2  LatchInput=off
  BC : Inport  Port=3  LatchInput=off
  CA : Inport  Port=4  LatchInput=off
  Freq : Inport  Port=5  LatchInput=off
  Block : Inport  Port=6  LatchInput=off
  6 Flip-Flop : Subsystem
  Data Type  Conversion : DataTypeConversion  Orientation=down  OutDataTypeMode=boolean  SaturateOnIntegerOverflow=on  RndMeth=Zero
  Data Type  Conversion1 : DataTypeConversion  OutDataTypeMode=boolean  SaturateOnIntegerOverflow=on  RndMeth=Zero
  Data Type  Conversion2 : DataTypeConversion  OutDataTypeMode=boolean  SaturateOnIntegerOverflow=on  RndMeth=Zero
  Data Type  Conversion3 : DataTypeConversion  OutDataTypeMode=boolean  SaturateOnIntegerOverflow=on  RndMeth=Zero
  Data Type  Conversion4 : DataTypeConversion  Orientation=down  OutDataTypeMode=double  SaturateOnIntegerOverflow=on  RndMeth=Zero
  Discrete-Time Integrator : DiscreteIntegrator  IntegratorMethod=Integration: Trapezoidal  ExternalReset=rising  SampleTime=Ts  ICPrevOutput=DiscIntNeverNeededParam  ICPrevScaledInput=DiscIntNeverNeededParam
  Discrete-Time Integrator1 : DiscreteIntegrator  IntegratorMethod=Integration: Trapezoidal  ExternalReset=rising  SampleTime=Ts  ICPrevOutput=DiscIntNeverNeededParam  ICPrevScaledInput=DiscIntNeverNeededParam
  Double Pulse : Switch  Threshold=0.5  InputSameDT=on
  Gain : Gain  Gain=-1  SaturateOnIntegerOverflow=on
  Gain1 : Gain  Gain=-1  SaturateOnIntegerOverflow=on
  Gain2 : Gain  Gain=-1  SaturateOnIntegerOverflow=on
  K2 : Constant  Value=Double_Pulse
  K3 : Constant  Value=0
  Logical Operator : Logic
  Logical Operator1 : Logic  Operator=OR
  Logical Operator2 : Logic  Orientation=left
  Logical Operator3 : Logic  Operator=NOT  Inputs=1
  Logical Operator5 : Logic  Orientation=left  Operator=NOT  Inputs=1
  Mux : Mux  Inputs=6
  Pwidth : Constant  Value=pwidth
  Relational Operator : RelationalOperator  InputSameDT=on
  Relational Operator1 : RelationalOperator  InputSameDT=on
  Relational Operator2 : RelationalOperator  Operator=<  InputSameDT=on
  Selector : Selector  Elements=[2 3 4 5 6 1 ]  InputPortWidth=6
  Talpha3 : Gain  Gain=1/360  SaturateOnIntegerOverflow=on
  Twidth1 : Gain  Gain=1/360  SaturateOnIntegerOverflow=on
  Unit Delay : UnitDelay  SampleTime=Ts
  pulses : Outport  InitialOutput=0
  wires:
  alpha_deg/1 -> Talpha3/1
  6 Flip-Flop/1(Q) -> Logical Operator5/1
  Freq/1 -> Discrete-Time Integrator1/1, Discrete-Time Integrator/1
  BC/1 -> Mux/2, Gain2/1
  CA/1 -> Mux/4, Gain/1
  Mux/1 -> Relational Operator/1
  Talpha3/1 -> Relational Operator1/2
  Logical Operator5/1 -> Logical Operator2/2
  Relational Operator/1 -> Discrete-Time Integrator/2, Data Type  Conversion1/1
  K3/1 -> Relational Operator/2
  Gain2/1 -> Mux/5
  Gain1/1 -> Mux/3
  Gain/1 -> Mux/1
  Discrete-Time Integrator/1 -> Relational Operator1/1  "RAMP"
  Discrete-Time Integrator1/1 -> Relational Operator2/1  "RAMP"
  Twidth1/1 -> Relational Operator2/2
  Pwidth/1 -> Twidth1/1
  Logical Operator1/1 -> Double Pulse/1
  Selector/1 -> Logical Operator1/2
  Logical Operator/1 -> Logical Operator1/1, Selector/1, Double Pulse/3, Unit Delay/1
  K2/1 -> Double Pulse/2
  Unit Delay/1 -> 6 Flip-Flop/1(S)
  Logical Operator3/1 -> Logical Operator/2
  AB/1 -> Gain1/1, Mux/6
  Logical Operator2/1 -> Discrete-Time Integrator1/2  "START_PULSE"
  Relational Operator1/1 -> Data Type  Conversion/1  "RAMP>alpha"
  Data Type  Conversion/1 -> Logical Operator2/1
  Data Type  Conversion1/1 -> 6 Flip-Flop/2(R)
  Relational Operator2/1 -> Data Type  Conversion2/1
  Data Type  Conversion2/1 -> Logical Operator/1
  Block/1 -> Data Type  Conversion3/1
  Data Type  Conversion3/1 -> Logical Operator3/1
  Double Pulse/1 -> Data Type  Conversion4/1
  Data Type  Conversion4/1 -> pulses/1

== system powerlib_extras/Discrete  Control Blocks/Discrete Variable Transport Delay ==
  In : Inport  Port=1  LatchInput=off
  D : Inport  Port=2  LatchInput=off
  "S-Function " : S-Function  FunctionName=discreteVariableTransportDelay  Parameters=MaxDelay,Ts,InitialValue
  Out : Outport
  wires:
  "S-Function "/1 -> Out/1
  In/1 -> "S-Function "/1
  D/1 -> "S-Function "/2

== system powerlib_extras/Measurements/3-Phase Sequence Analyzer ==
  note: Zero sequence :V0 = 1/3 * (Va + Vb + Vc )
  note: where a =exp(j *2pi/3) = 1 < + 120 deg.
  note: Positive sequence :V1 = 1/3 * (Va + a*Vb + a^2 *Vc )
  note: Negative sequence :V2 = 1/3 * (Va + a^2*Vb + a *Vc )
  abc : Inport  Port=1  PortDimensions=3  LatchInput=off
  Complex to Magnitude-Angle : ComplexToMagnitudeAngle
  Constant : Constant  Value=PosOn
  Constant1 : Constant  Value=NegOn
  Constant2 : Constant  Value=ZeroOn
  Demux : Demux  Outputs=3
  Determine if pha20 are set to zero : Subsystem
  Mux : Mux  Inputs=3
  Mux1 : Mux  Inputs=3
  Neg. Seq. Computation : Subsystem  TreatAsAtomicUnit=on
  PhasorA : Subsystem
  PhasorB : Subsystem
  PhasorC : Subsystem
  Pos. Seq. Computation : Subsystem  TreatAsAtomicUnit=on
  Selector : Selector  Elements=SelectElement  InputPortWidth=3
  Selector1 : Selector  Elements=SelectElement  InputPortWidth=3
  Zero Seq. Computation : Subsystem  TreatAsAtomicUnit=on
  cos(nwt) : Sin  Frequency=2*pi*n*f1  Phase=pi/2  SampleTime=0
  rad->deg1 : Gain  Gain=180/pi  SaturateOnIntegerOverflow=on
  sin(nwt) : Sin  Frequency=2*pi*n*f1  SampleTime=0
  Mag : Outport  InitialOutput=0
  Phase : Outport  Port=2  InitialOutput=0
  wires:
  PhasorC/1(Out) -> Mux/3
  PhasorB/1(Out) -> Mux/2
  PhasorA/1(Out) -> Mux/1
  rad->deg1/1 -> Phase/1
  Mux/1 -> Pos. Seq. Computation/1(In), Neg. Seq. Computation/1(In), Zero Seq. Computation/1(In)
  Pos. Seq. Computation/1(Out) -> Mux1/1
  Neg. Seq. Computation/1(Out) -> Mux1/2
  Zero Seq. Computation/1(Out) -> Mux1/3
  Mux1/1 -> Complex to Magnitude-Angle/1
  Complex to Magnitude-Angle/1 -> Determine if pha20 are set to zero/1(Mag120), Selector/1
  Constant/1 -> Pos. Seq. Computation/Enable
  Constant2/1 -> Zero Seq. Computation/Enable
  Selector/1 -> Mag/1
  Determine if pha20 are set to zero/1(Pha120) -> Selector1/1
  Selector1/1 -> rad->deg1/1
  Constant1/1 -> Neg. Seq. Computation/Enable
  Complex to Magnitude-Angle/2 -> Determine if pha20 are set to zero/2(Pha120*)
  cos(nwt)/1 -> PhasorC/3(cos), PhasorB/3(cos), PhasorA/3(cos)
  sin(nwt)/1 -> PhasorC/2(sin), PhasorB/2(sin), PhasorA/2(sin)
  Demux/3 -> PhasorC/1(in)
  Demux/2 -> PhasorB/1(in)
  abc/1 -> Demux/1
  Demux/1 -> PhasorA/1(in)

== system powerlib_extras/Measurements/3-phase  Instantaneous  Active & Reactive Power ==
  note: Gilbert Sybille, Pierre Giroux
      | Power System Simulation Laboratory
      | IREQ, Hydro-Quebc
  note: 3-phase instantaneous active and reactive power
  note: Note: Equation 2 is valid only for a balanced and harmonic-free system.
  note: This block computes the 3-phase instantaneous real power and reactive power using the following equations:
  note: 2) Q = 1/sqrt(3)* (Vbc*Ia + Vca*Ib + Vab*Ic)
  note: 1) P = Va*Ia + Vb*Ib + Vc*Ic
  Vabc : Inport  Port=1  PortDimensions=3  LatchInput=off
  Iabc : Inport  Port=2  PortDimensions=3  LatchInput=off
  Demux : Demux  Outputs=3
  Mux : Mux  Inputs=3
  Mux1 : Mux  Inputs=2
  Product1 : Product  SaturateOnIntegerOverflow=on  InputSameDT=on
  Product3 : Product  SaturateOnIntegerOverflow=on  InputSameDT=on
  Sum : Sum  Inputs=+-  SaturateOnIntegerOverflow=on  InputSameDT=on
  Sum1 : Sum  Inputs=1  SaturateOnIntegerOverflow=on  InputSameDT=on
  Sum4 : Sum  Inputs=1  SaturateOnIntegerOverflow=on  InputSameDT=on
  Sum5 : Sum  Inputs=+-  SaturateOnIntegerOverflow=on  InputSameDT=on
  Sum6 : Sum  Inputs=+-  SaturateOnIntegerOverflow=on  InputSameDT=on
  pu->V : Gain  Gain=1/sqrt(3)  SaturateOnIntegerOverflow=on
  PQ : Outport
  wires:
  Mux1/1 -> PQ/1
  pu->V/1 -> Mux1/2  "Q"
  Mux/1 -> Product3/1
  Sum6/1 -> Mux/2
  Sum5/1 -> Mux/1
  Sum/1 -> Mux/3
  Demux/3 -> Sum6/1, Sum5/2
  Demux/2 -> Sum5/1, Sum/2
  Demux/1 -> Sum6/2, Sum/1
  Sum4/1 -> Mux1/1  "P"
  Iabc/1 -> Product3/2, Product1/2
  Vabc/1 -> Demux/1, Product1/1
  Product1/1 -> Sum4/1
  Product3/1 -> Sum1/1
  Sum1/1 -> pu->V/1

== system powerlib_extras/Measurements/Active & Reactive Power ==
  V : Inport  Port=1  LatchInput=off
  I : Inport  Port=2  LatchInput=off
  Deg->Rad : Gain  Gain=pi/180  SaturateOnIntegerOverflow=on
  Gain : Gain  Gain=1/2  SaturateOnIntegerOverflow=on
  I_Fundamental : powerlib_extras/Measurements/Fourier  f1=f1  n=1
  Mux1 : Mux  Inputs=2
  Product : Product  SaturateOnIntegerOverflow=on  InputSameDT=on
  Product1 : Product  SaturateOnIntegerOverflow=on  InputSameDT=on
  Product2 : Product  SaturateOnIntegerOverflow=on  InputSameDT=on
  Sum : Sum  Inputs=+-  SaturateOnIntegerOverflow=on  InputSameDT=on
  Trigonometric Function : Trigonometry
  Trigonometric Function1 : Trigonometry  Operator=cos
  V_Fundamental : powerlib_extras/Measurements/Fourier  f1=f1  n=1
  PQ : Outport  InitialOutput=0
  wires:
  I_Fundamental/2 -> Sum/2
  V_Fundamental/2 -> Sum/1
  I_Fundamental/1 -> Product/2
  V_Fundamental/1 -> Product/1
  Sum/1 -> Deg->Rad/1
  Deg->Rad/1 -> Trigonometric Function/1, Trigonometric Function1/1
  Trigonometric Function/1 -> Product2/2
  Product/1 -> Product2/1, Product1/1
  Trigonometric Function1/1 -> Product1/2
  Product1/1 -> Mux1/1
  Product2/1 -> Mux1/2
  Mux1/1 -> Gain/1
  Gain/1 -> PQ/1
  V/1 -> V_Fundamental/1
  I/1 -> I_Fundamental/1

== system powerlib_extras/Measurements/Fourier ==
  signal : Inport  Port=1  LatchInput=off
  Fcn : Fcn  Expr=u^2
  Fcn1 : Fcn  Expr=u^2
  Fcn2 : Fcn  Expr=sqrt(u)
  Fcn3 : Fcn  Expr=180/pi*atan2(u[2],u[1])
  Gain1 : Gain  Gain=k*f1  SaturateOnIntegerOverflow=on
  Integ2 : Integrator
  Mux : Mux  Inputs=2
  Product : Product  SaturateOnIntegerOverflow=on  InputSameDT=on
  Product1 : Product  SaturateOnIntegerOverflow=on  InputSameDT=on
  Sum : Sum  SaturateOnIntegerOverflow=on  InputSameDT=on
  Sum1 : Sum  Inputs=+-  SaturateOnIntegerOverflow=on  InputSameDT=on
  Sum2 : Sum  Inputs=+-  SaturateOnIntegerOverflow=on  InputSameDT=on
  T : TransportDelay  DelayTime=1/f1  BufferSize=2048
  T1 : TransportDelay  DelayTime=1/f1  BufferSize=2048
  cos(nwt) : Sin  Frequency=2*pi*n*f1  Phase=pi/2  SampleTime=0
  integ1 : Integrator
  sin(nwt) : Sin  Frequency=2*pi*n*f1  SampleTime=0
  magnitude : Outport  InitialOutput=0
  angle : Outport  Port=2  InitialOutput=0
  wires:
  Sum/1 -> Fcn2/1
  Fcn/1 -> Sum/1
  Fcn1/1 -> Sum/2
  Mux/1 -> Fcn3/1
  Fcn3/1 -> angle/1
  sin(nwt)/1 -> Product/1
  cos(nwt)/1 -> Product1/2
  Product/1 -> integ1/1
  Product1/1 -> Integ2/1
  T/1 -> Sum1/2
  T1/1 -> Sum2/2
  integ1/1 -> Sum1/1, T/1
  Integ2/1 -> Sum2/1, T1/1
  Sum2/1 -> Fcn1/1, Mux/2
  Sum1/1 -> Fcn/1, Mux/1
  signal/1 -> Gain1/1
  Gain1/1 -> Product/2, Product1/1
  Fcn2/1 -> magnitude/1

== system powerlib_extras/Measurements/Mean Value ==
  note: Mean value
  In : Inport  Port=1  LatchInput=off
  Gain : Gain  Gain=1/Period  SaturateOnIntegerOverflow=on
  Sum : Sum  Inputs=+-  SaturateOnIntegerOverflow=on  InputSameDT=on
  Transport Delay : TransportDelay  DelayTime=Period
  integrator : Integrator
  Mean : Outport
  wires:
  Transport Delay/1 -> Sum/2
  integrator/1 -> Transport Delay/1, Sum/1
  In/1 -> integrator/1
  Sum/1 -> Gain/1
  Gain/1 -> Mean/1

== system powerlib_extras/Measurements/Mean Value (linear) ==
  note: |
      | |
      | |
      | |
      | |
      | |
      | |
  note: __________________________________________________________________
  note: * In
  note: Out =
  note: Implements the following expression
      | (using the Pade fonction):
  note: T * s
  note: __________
  note: 1 - exp(-T*s)
  In : Inport  Port=1  LatchInput=off
  Gain1 : Gain  Gain=Freq  SaturateOnIntegerOverflow=on
  Integrator : Integrator  InitialCondition=Vinit
  Pade approximation of 1 cycle delay : StateSpace  A=Ac  B=Bc  C=Cc  D=Dc  X0=x0c
  Sum : Sum  Inputs=|+-  SaturateOnIntegerOverflow=on
  Mean : Outport
  wires:
  Sum/1 -> Gain1/1
  Pade approximation of 1 cycle delay/1 -> Sum/2
  In/1 -> Pade approximation of 1 cycle delay/1, Sum/1
  Gain1/1 -> Integrator/1
  Integrator/1 -> Mean/1  "Mean value"

== system powerlib_extras/Measurements/RMS ==
  signal : Inport  Port=1  LatchInput=off
  Abs : Abs  SaturateOnIntegerOverflow=on
  Gain : Gain  Gain=f1  SaturateOnIntegerOverflow=on
  Math Function : Math  Operator=square  SaturateOnIntegerOverflow=on
  Math Function1 : Math  Operator=sqrt  SaturateOnIntegerOverflow=on
  Sum1 : Sum  Inputs=+-  SaturateOnIntegerOverflow=on  InputSameDT=on
  T : TransportDelay  DelayTime=1/f1
  integ : Integrator
  rms : Outport  InitialOutput=0
  wires:
  Abs/1 -> Math Function1/1
  Sum1/1 -> Abs/1
  T/1 -> Sum1/2
  integ/1 -> T/1, Sum1/1
  Math Function1/1 -> rms/1
  signal/1 -> Math Function/1
  Math Function/1 -> Gain/1
  Gain/1 -> integ/1

== system powerlib_extras/Measurements/Total Harmonic Distorsion ==
  note: THD= Uhrms /U1rms
      |
      | where:
      |
      | Uhrms =  rms value of harmonics = sqrt( U2^2 + U3^2 + U4^2....) =  sqrt( Urms^2 -U1rms^2)
      | U1rms =  rms value of the fundamenrtal component
      | Urms = true rms value including harmonics
  signal : Inport  Port=1  LatchInput=off
  Constant : Constant  Value=eps
  Fourier fundamental : powerlib_extras/Measurements/Fourier  f1=f1  n=1
  Math Function : Math  Operator=square  SaturateOnIntegerOverflow=on
  Math Function2 : Math  Operator=sqrt  SaturateOnIntegerOverflow=on
  Math Funtion1 : Math  Operator=square  SaturateOnIntegerOverflow=on
  Product : Product  Inputs=*/  SaturateOnIntegerOverflow=on  InputSameDT=on
  RMS : powerlib_extras/Measurements/RMS  f1=f1
  Sum : Sum  Inputs=+-  SaturateOnIntegerOverflow=on  InputSameDT=on
  Sum1 : Sum  Inputs=+-  SaturateOnIntegerOverflow=on  InputSameDT=on
  Terminator : Terminator
  peak to rms : Gain  Gain=1/sqrt(2)  SaturateOnIntegerOverflow=on
  THD : Outport
  wires:
  Fourier fundamental/2 -> Terminator/1
  Constant/1 -> Sum1/2
  peak to rms/1 -> Sum1/1, Math Funtion1/1  "U1 rms"
  Sum1/1 -> Product/2
  Fourier fundamental/1 -> peak to rms/1
  RMS/1 -> Math Function/1  "U rms"
  Product/1 -> THD/1
  Math Function2/1 -> Product/1  "Uhrms"
  Math Funtion1/1 -> Sum/2
  Sum/1 -> Math Function2/1
  Math Function/1 -> Sum/1
  signal/1 -> Fourier fundamental/1, RMS/1

== system powerlib_extras/Measurements/abc_to_dq0 Transformation ==
  note: Vq= 2/3 (Va*coswt + Vb*cos(wt-2pi/3) + Vc*cos(wt+2pi/3)
  note: Vd= 2/3 (Va*sinwt + Vb*sin(wt-2pi/3) + Vc*sin(wt+2pi/3)
  note: V0= 1/3 (Va + Vb + Vc )
  abc : Inport  Port=1  PortDimensions=3  LatchInput=off
  sin_cos : Inport  Port=2  PortDimensions=2  LatchInput=off
  Demux : Demux  Outputs=2
  Fcn1 : Fcn  Expr=2/3*((u[1]*u[5])+(u[2]*u[7])+(u[3]*u[9]))
  Fcn2 : Fcn  Expr=2/3*((u[1]*u[4])+(u[2]*u[6])+(u[3]*u[8]))
  Gain1 : Gain  Gain=1/3  SaturateOnIntegerOverflow=on
  K1 : Constant  Value=0.5
  K2 : Constant  Value=sqrt(3)/2
  Mux : Mux  Inputs=2
  Mux1 : Mux  Inputs=3
  Mux2 : Mux  Inputs=6
  Product{,1..3} (4 alike) : Product  SaturateOnIntegerOverflow=on  InputSameDT=on
  Sum : Sum  Inputs=--  SaturateOnIntegerOverflow=on  InputSameDT=on
  Sum1 : Sum  Inputs=-+  SaturateOnIntegerOverflow=on  InputSameDT=on
  Sum2 : Sum  Inputs=--  SaturateOnIntegerOverflow=on  InputSameDT=on
  Sum3 : Sum  Inputs=--  SaturateOnIntegerOverflow=on  InputSameDT=on
  Sum4 : Sum  Inputs=1  SaturateOnIntegerOverflow=on  InputSameDT=on
  dq0 : Outport  InitialOutput=0
  wires:
  abc/1 -> Mux/1  "Vabc"
  Mux2/1 -> Mux/2
  sin_cos/1 -> Demux/1
  Demux/2 -> Sum3/2, Product3/1, Product1/1, Mux2/2  "cos(wt)"
  Demux/1 -> Product/1, Product2/1, Sum2/2, Mux2/1  "sin(wt)"
  Product/1 -> Sum/1
  Product1/1 -> Sum/2
  Product3/1 -> Sum1/1
  Product2/1 -> Sum1/2
  Sum3/1 -> Mux2/6  "cos(wt+2pi/3)"
  Sum2/1 -> Mux2/5  "sin(wt+2pi/3)"
  K1/1 -> Product/2, Product3/2
  K2/1 -> Product1/2, Product2/2
  Sum/1 -> Mux2/3, Sum2/1  "sin(wt-2pi/3)"
  Sum1/1 -> Mux2/4, Sum3/1  "cos(wt-2pi/3)"
  Mux/1 -> Fcn2/1, Fcn1/1, Sum4/1
  Sum4/1 -> Gain1/1
  Mux1/1 -> dq0/1
  Fcn1/1 -> Mux1/2  "Vq"
  Fcn2/1 -> Mux1/1  "Vd"
  Gain1/1 -> Mux1/3
